simulink model "fam_force_allocation_module_hrn"  (R2015b)
settings: Solver=ode3  StartTime=0.0  StopTime=sim_stop_time  FixedStep=astrobee_time_step_size  RelTol=1e-3
libraries: simulink x1, fam_force_allocation_module_lib x1
settings Model: PauseTimes=15  Creator=jfusco1  LastModifiedBy=rhnakamu
settings DataIOCC: SaveFormat=Array
settings DebuggingCC: SolverPrmCheckMsg=warning
settings HardwareCC: ProdBitPerPointer=32  ProdLargestAtomicFloat=None  ProdIntDivRoundTo=Undefined  ProdEndianess=Unspecified  ProdWordSize=32  ProdHWDeviceType=32-bit Generic
settings GRTTargetCC: GeneratePreprocessorConditionals=Disable all
settings ConfigComp: CovModelRefEnable=Off  CovSFcnEnable=off

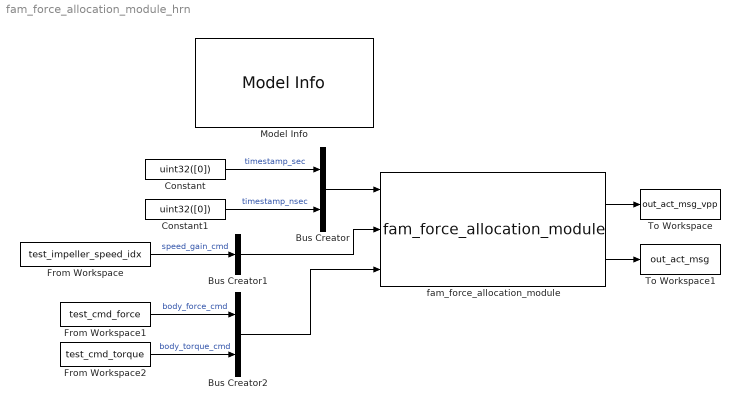
== system fam_force_allocation_module_hrn ==
  Bus Creator : BusCreator  Inputs=2
  Bus Creator1 : BusCreator  Inputs=1
  Bus Creator2 : BusCreator  Inputs=2
  Constant : Constant  Value=uint32([0])
  Constant1 : Constant  Value=uint32([0])
  From Workspace : FromWorkspace  VariableName=test_impeller_speed_idx  SampleTime=0  Interpolate=off  OutputAfterFinalValue=Holding final value
  From Workspace1 : FromWorkspace  VariableName=test_cmd_force  SampleTime=0  Interpolate=off  OutputAfterFinalValue=Holding final value
  From Workspace2 : FromWorkspace  VariableName=test_cmd_torque  SampleTime=0  Interpolate=off  OutputAfterFinalValue=Holding final value
  Model Info : simulink/Model-Wide Utilities/Model Info  Frame=on  DisplayStringWithTags=|  HorizontalTextAlignment=Left  LeftAlignmentValue=0.02  SourceBlockDiagram=fam_force_allocation_module_hrn  TagMaxNumber=20
      | Force Allocation Module Harness
      | Created: %<Created>
      | By: %<Creator>
      | 
      | Last Modified by: %<ModifiedBy>
      | On: %<ModifiedDate>
  To Workspace : ToWorkspace  VariableName=out_act_msg_vpp  SaveFormat=Timeseries  SampleTime=-1
  To Workspace1 : ToWorkspace  VariableName=out_act_msg  SaveFormat=Timeseries  SampleTime=-1
  fam_force_allocation_module : fam_force_allocation_module_lib/fam_force_allocation_module
  wires:
  fam_force_allocation_module/1 -> To Workspace/1
  fam_force_allocation_module/2 -> To Workspace1/1
  Constant/1 -> Bus Creator/1  "timestamp_sec"
  Constant1/1 -> Bus Creator/2  "timestamp_nsec"
  Bus Creator/1 -> fam_force_allocation_module/1
  Bus Creator1/1 -> fam_force_allocation_module/2
  From Workspace/1 -> Bus Creator1/1  "speed_gain_cmd"
  Bus Creator2/1 -> fam_force_allocation_module/3
  From Workspace1/1 -> Bus Creator2/1  "body_force_cmd"
  From Workspace2/1 -> Bus Creator2/2  "body_torque_cmd"
